simulink model "rsimtfdemo"  (Simulink 6.0)
settings: Solver=ode2  SolverMode=SingleTasking  StartTime=0.0  StopTime=1.0  FixedStep=.001  RelTol=1e-3
undefined symbols (not defined in the file or in its folder): w, zeta
settings Model: Creator=jims  LastModifiedBy=pszpak  ExtModeTrigMode=oneshot  ExtModeArmWhenConnect=off  ExtModeAutoUpdateStatusClock=off  ProdHWDeviceType=Specified
settings DataIOCC: LimitDataPoints=off  SignalLoggingName=sigsOut
settings OptimizationCC: BlockReduction=off  BooleanDataType=off  InlineInvariantSignals=off
settings DebuggingCC: CheckExecutionContextPreStartOutputMsg=on  CheckExecutionContextRuntimeOutputMsg=on  SolverPrmCheckMsg=none
settings HardwareCC: ProdBitPerShort=32  ProdBitPerInt=16  ProdHWDeviceType=Specified  TargetHWDeviceType=MATLAB Host  ProdEqTarget=off
settings RTWCC: SystemTargetFile=rsim.tlc  TLCOptions=-p0  TemplateMakefile=rsim_default_tmf  RetainRTWFile=on  ProcessScript=rsim_make_rtw_hook
settings CodeAppCC: PrefixModelToSubsysFcnNames=off
settings RSimTargetCC: TargetFcnLib=ansi_tfl_tmw.mat  GenFloatMathFcnCalls=ANSI_C  IsPILTarget=off

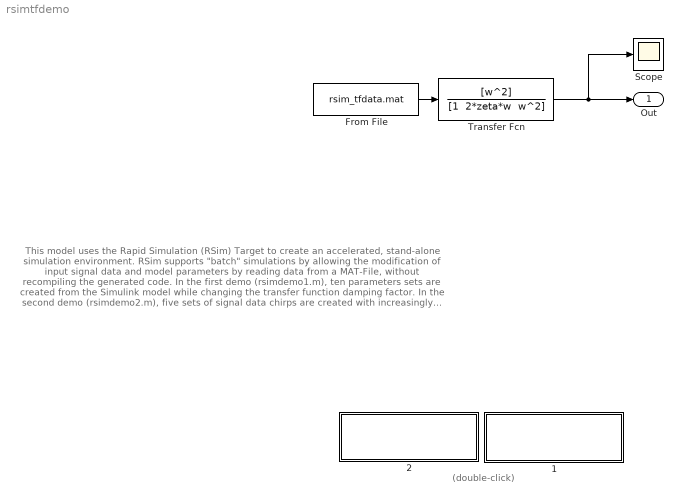
== system rsimtfdemo ==
  note: This model uses the Rapid Simulation (RSim) Target to create an accelerated,
      | stand-alone simulation environment.  RSim supports "batch" simulations by allowing
      | the modification of input signal data and model parameters by reading data from a
      | MAT-File, without recompiling the generated code.
      |
      | In the first demo (rsimdemo1.m), ten parameters sets are created from the Simulink model
      | while changing the transfer function damping factor. In the second demo (rsimdemo2.m),
      | five sets of signal data chirps are created with increasingly higher frequencies.  In each
      | demo, the RSim executable runs the set of simulations and creates output MAT-Files
      | containing the specific simulation result. In the end, a composite for all runs is plotted
      | in a MATLAB figure.
      |
      | Note that RSIM also supports variable step solvers.  For more information, refer to the
      | "Rapid Simulation Target" chapter in the Real-Time Workshop User's Guide.
  note: (double-click)
  " 1" : Subsystem  PropExecContextAcrossSSBoundary=on
      settings: OpenFcn=rsimdemo2;
      mask Display: disp('Run second demo\n(rsimdemo2.m)')
  " 2" : Subsystem  PropExecContextAcrossSSBoundary=on
      settings: OpenFcn=rsimdemo1;
      mask Display: disp('Run first demo\n(rsimdemo1.m)')
  From File : FromFile  FileName=rsim_tfdata.mat  SampleTime=0
  Scope : Scope
  Transfer Fcn : TransferFcn  Numerator=[w^2]  Denominator="[1  2*zeta*w  w^2]"
  Out : Outport
  wires:
  From File/1 -> Transfer Fcn/1
  Transfer Fcn/1 -> Out/1, Scope/1

== system rsimtfdemo/ 1 ==

== system rsimtfdemo/ 2 ==
